simulink subsystem "Subsystem_Obstaculos_Leds"  (R2023b)
settings: Solver=VariableStepAuto  StartTime=0.0  StopTime=10.0  RelTol=1e-3
libraries: simulink x3
settings Model: Creator=Alberto  LastModifiedBy=Alberto

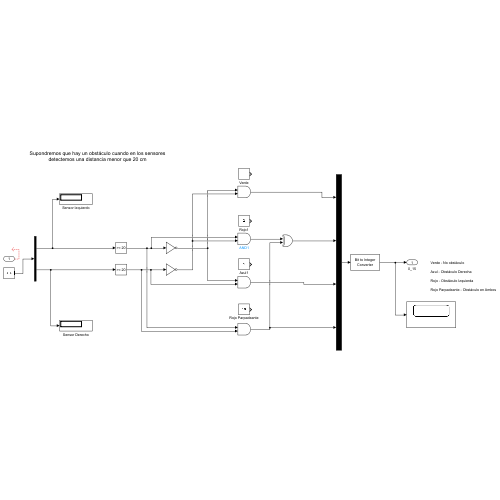
[thumbnail: Simulink's stored preview of the top-level diagram]
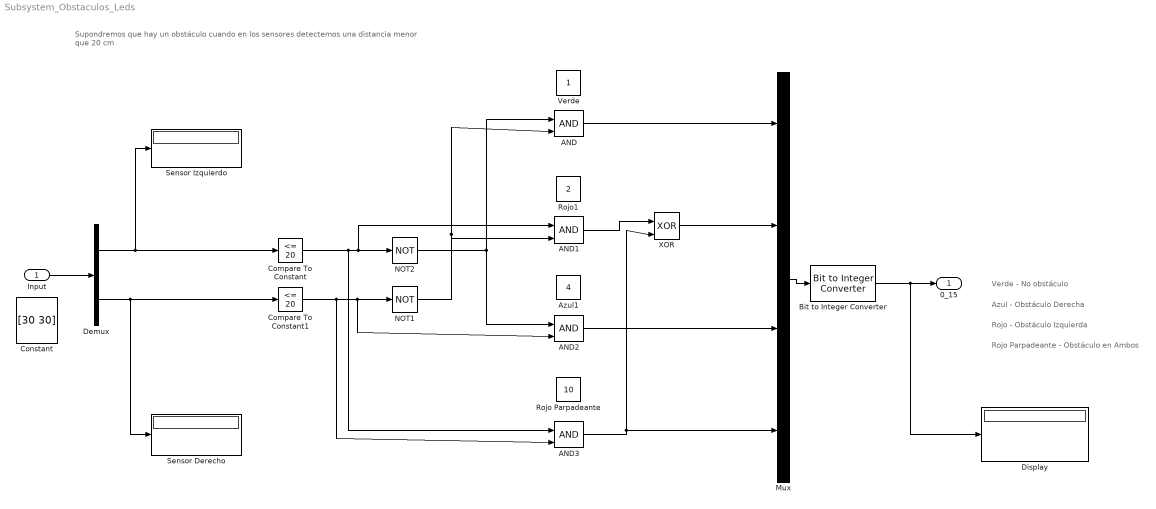
== system Subsystem_Obstaculos_Leds ==
  note: Verde - No obstáculo
  note: Azul - Obstáculo Derecha
  note: Rojo - Obstáculo Izquierda
  note: Rojo Parpadeante - Obstáculo en Ambos
  note: Supondremos que hay un obstáculo cuando en los sensores detectemos una distancia menor que 20 cm
  Input : Inport
  AND{,1..3} (4 alike) : Logic  IconShape=distinctive  AllPortsSameDT=off  OutDataTypeStr=boolean
  Azul1 : Constant  Value=4
  Bit to Integer Converter : simulink/Logic and Bit Operations/Bit to Integer Converter  nbits=4  bitOrder=LSB first  signedOutputValues=Unsigned  outDtype=Inherit via internal rule  outDtypeSigned=Inherit via internal rule
  Compare To Constant : simulink/Logic and Bit Operations/Compare To Constant  relop=<=  const=20  OutDataTypeStr=boolean
  Compare To Constant1 : simulink/Logic and Bit Operations/Compare To Constant  relop=<=  const=20  OutDataTypeStr=boolean
  Constant : Constant  Value=[30 30]
  Demux : Demux  Outputs=2
  Display : Display
  Mux : Mux
  NOT1 : Logic  Operator=NOT  IconShape=distinctive  AllPortsSameDT=off  OutDataTypeStr=boolean
  NOT2 : Logic  Operator=NOT  IconShape=distinctive  AllPortsSameDT=off  OutDataTypeStr=boolean
  Rojo Parpadeante : Constant  Value=10
  Rojo1 : Constant  Value=2
  Sensor Derecho : Display
  Sensor Izquierdo : Display
  Verde : Constant
  XOR : Logic  Operator=XOR  IconShape=distinctive  AllPortsSameDT=off  OutDataTypeStr=boolean
  0_15 : Outport
  wires:
  Demux/2 -> Compare To Constant1/1, Sensor Derecho/1
  Demux/1 -> Compare To Constant/1, Sensor Izquierdo/1
  Compare To Constant/1 -> AND3/1, AND1/1, NOT2/1
  Compare To Constant1/1 -> AND3/2, AND2/2, NOT1/1
  XOR/1 -> Mux/2
  AND3/1 -> Mux/4, XOR/2
  AND1/1 -> XOR/1
  NOT2/1 -> AND2/1, AND/1
  NOT1/1 -> AND1/2, AND/2
  Mux/1 -> Bit to Integer Converter/1
  Bit to Integer Converter/1 -> 0_15/1, Display/1
  AND/1 -> Mux/1
  AND2/1 -> Mux/3
  Input/1 -> Demux/1
